simulink model "simulateController"  (R2022a)
settings: Solver=ode5  StartTime=0.0  StopTime=480  RelTol=1e-3
values from neighbouring files (symbols this model uses):
  ss_d = c2d(bicycle, opts.Ts_mpc)    [readySimulation.m]
undefined symbols (not defined in the file or in its folder): A_full, B_full, C_full, lb_u_full, lb_x_full, opts, QstructInitial, R_full, R_full_zeros, ub_u_full, ub_x_full
settings Model: PacingRate=0.350000  Creator=simonas  LastModifiedBy=simonas
settings HardwareCC: ProdBitPerLong=64  ProdHWDeviceType=Intel->x86-64 (Linux 64)
settings RTWCC: Description=Simulink Desktop Real-Time  SystemTargetFile=sldrt.tlc  TemplateMakefile=sldrt.tmf  RTWCompilerOptimization=on
settings CodeAppCC: MaxIdLength=95
settings SimulinkDesktopRealTimeCC: TargetLibSuffix=_sldrt.a  TargetPreCompLibLocation=C:\Program Files\MATLAB\R2022a\toolbox\sldrt\lib\win64

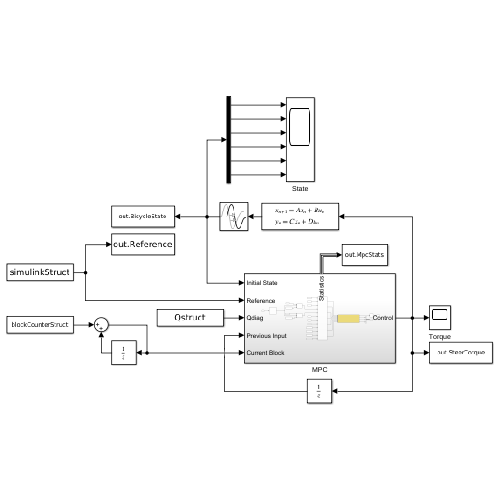
[thumbnail: Simulink's stored preview of the top-level diagram]
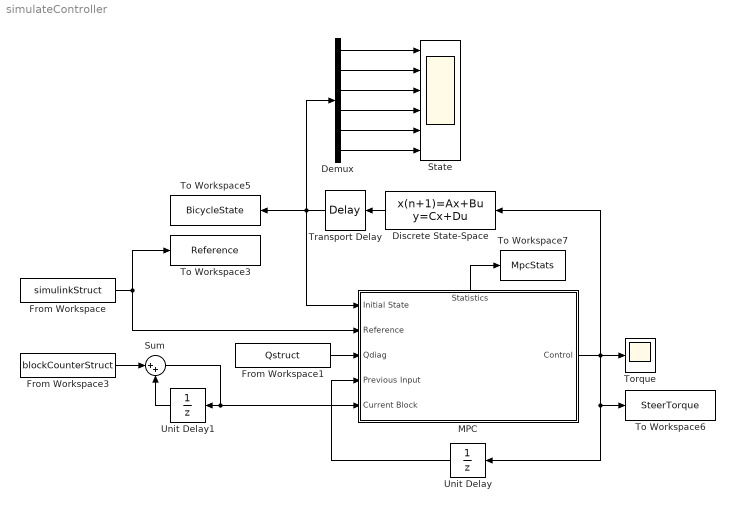
== system simulateController ==
  Demux : Demux  Outputs=6
  Discrete State-Space : DiscreteStateSpace  A=ss_d.A  B=ss_d.B  C=ss_d.C  D=ss_d.D  InitialCondition=[0; 0; 0; 0; 0; 0]  SampleTime=-1
  From Workspace : FromWorkspace  VariableName=simulinkStruct  SampleTime=opts.Ts_mpc  Interpolate=off  OutputAfterFinalValue=Cyclic repetition
  From Workspace1 : FromWorkspace  VariableName=Qstruct  SampleTime=opts.Ts_mpc  Interpolate=off  OutputAfterFinalValue=Cyclic repetition
  From Workspace3 : FromWorkspace  VariableName=blockCounterStruct  SampleTime=opts.Ts_mpc  Interpolate=off  OutputAfterFinalValue=Cyclic repetition
  MPC : Subsystem
      settings: PortSchema="{\"entries\":[{\"content\":{\"sides\":[{\"content\":{\"connectorIds\":[\"In1\",\"In2\",\"In3\",\"In4\",\"In5\"]},\"type\":\"ConnectorPlacement.EquallySpacedRectSide\",\"uuid\":\"837940b0-492f-49e7-ad78-2f53a96cfdb0\"},{\"content\":{\"connectorIds\":[\"Out1\"],\"side\":\"RIGHT\"},\"type\":\"ConnectorPlacement.EquallySpacedRectSide\",\"uuid\":\"0b454771-57c7-4798-97e4-6e41a25b36dc\"},{\"content\":{\"connectorIds\":[\"Out2\"],\"side\":\"TOP\"},\"type\":\"ConnectorPlacement.EquallySpacedRectSide\",\"uuid\":\"d0d77e63-f0c6-441e-9a4a-b6dfb0057ad2\"},{\"content\":{\"connectorIds\":[],\"side\":\"BOTTOM\"},\"type\":\"ConnectorPlacement.EquallySpacedRectSide\",\"uuid\":\"b6921f02-8dc3-4ff1-8cb0-61ac83bc5ab1\"}]},\"type\":\"ConnectorPlacement.EquallySpacedConnector\",\"uuid\":\"6905a0a5-9fd3-4ab9-9143-61679843e617\"}],\"packageUris\":[\"http://schema.mathworks.com/mf0/Connector/R2020b\"],\"version\":\"1.0\"}"
  State : Scope  NumInputPorts=6
  Sum : Sum  Inputs=|++
  To Workspace3 : ToWorkspace  VariableName=Reference  SaveFormat=Timeseries  SampleTime=-1
  To Workspace5 : ToWorkspace  VariableName=BicycleState  SaveFormat=Timeseries  SampleTime=-1
  To Workspace6 : ToWorkspace  VariableName=SteerTorque  SaveFormat=Timeseries  SampleTime=-1
  To Workspace7 : ToWorkspace  VariableName=MpcStats  SaveFormat=Timeseries  SampleTime=-1
  Torque : Scope
  Transport Delay : TransportDelay  DelayTime=0.1  InitialOutput=[0; 0; 0; 0; 0; 0]
  Unit Delay : UnitDelay  SampleTime=opts.Ts_mpc  HasFrameUpgradeWarning=on
  Unit Delay1 : UnitDelay  InitialCondition=1  SampleTime=opts.Ts_mpc  HasFrameUpgradeWarning=on
  wires:
  Discrete State-Space/1 -> Transport Delay/1
  MPC/1(Control) -> To Workspace6/1, Unit Delay/1, Torque/1, Discrete State-Space/1
  From Workspace/1 -> To Workspace3/1, MPC/2(Reference)
  From Workspace1/1 -> MPC/3(Qdiag)
  MPC/2(Statistics) -> To Workspace7/1
  Unit Delay/1 -> MPC/4(Previous Input)
  Demux/1 -> State/1
  Demux/3 -> State/3
  Demux/4 -> State/4
  Demux/2 -> State/2
  Demux/5 -> State/5
  Demux/6 -> State/6
  Sum/1 -> MPC/5(Current Block), Unit Delay1/1
  Transport Delay/1 -> Demux/1, To Workspace5/1, MPC/1(Initial State)
  From Workspace3/1 -> Sum/1
  Unit Delay1/1 -> Sum/2

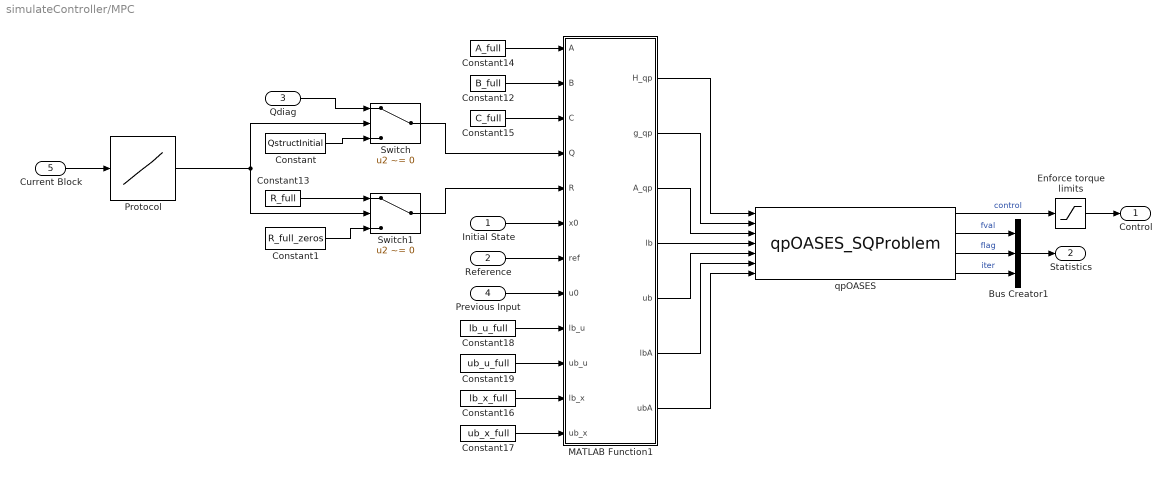
== system simulateController/MPC ==
  Initial State : Inport
  Reference : Inport  Port=2
  Qdiag : Inport  Port=3
  Previous Input : Inport  Port=4
  Current Block : Inport  Port=5
  Bus Creator1 : BusCreator  Inputs=3
  Constant : Constant  Value=QstructInitial
  Constant1 : Constant  Value=R_full_zeros  SampleTime=opts.Ts_mpc
  Constant12 : Constant  Value=B_full  SampleTime=opts.Ts_mpc
  Constant13 : Constant  Value=R_full  SampleTime=opts.Ts_mpc
  Constant14 : Constant  Value=A_full  SampleTime=opts.Ts_mpc
  Constant15 : Constant  Value=C_full  SampleTime=opts.Ts_mpc
  Constant16 : Constant  Value=lb_x_full  SampleTime=opts.Ts_mpc
  Constant17 : Constant  Value=ub_x_full  SampleTime=opts.Ts_mpc
  Constant18 : Constant  Value=lb_u_full  SampleTime=opts.Ts_mpc
  Constant19 : Constant  Value=ub_u_full  SampleTime=opts.Ts_mpc
  Enforce torque limits : Saturate  UpperLimit=opts.steerTorqueLim  LowerLimit=-opts.steerTorqueLim
  MATLAB Function1 : MATLAB Function  TreatAsAtomicUnit=on  SystemSampleTime=opts.Ts_mpc  VariantControl=Choice
  Protocol : Lookup_n-D  NumberOfTableDimensions=1  BreakpointsForDimension1=opts.lookupBreakpoints  Table=opts.lookupValues  InternalRulePriority=Speed  RndMeth=Simplest
  Switch : Switch  Criteria=u2 ~= 0  SaturateOnIntegerOverflow=off  InputSameDT=off
  Switch1 : Switch  Criteria=u2 ~= 0  SaturateOnIntegerOverflow=off  InputSameDT=off
  qpOASES : S-Function  FunctionName=qpOASES_SQProblem  SFunctionDeploymentMode=off  EnableBusSupport=off
  Control : Outport
  Statistics : Outport  Port=2
  wires:
  Enforce torque limits/1 -> Control/1
  Constant12/1 -> MATLAB Function1/2(B)
  Constant18/1 -> MATLAB Function1/9(lb_u)
  MATLAB Function1/1(H_qp) -> qpOASES/1
  Constant16/1 -> MATLAB Function1/11(lb_x)
  Constant19/1 -> MATLAB Function1/10(ub_u)
  Constant17/1 -> MATLAB Function1/12(ub_x)
  Bus Creator1/1 -> Statistics/1
  qpOASES/4 -> Bus Creator1/3  "iter"
  qpOASES/2 -> Bus Creator1/1  "fval"
  MATLAB Function1/3(A_qp) -> qpOASES/3
  Reference/1 -> MATLAB Function1/7(ref)
  qpOASES/3 -> Bus Creator1/2  "flag"
  MATLAB Function1/4(lb) -> qpOASES/4
  MATLAB Function1/2(g_qp) -> qpOASES/2
  Constant14/1 -> MATLAB Function1/1(A)
  MATLAB Function1/5(ub) -> qpOASES/5
  MATLAB Function1/7(ubA) -> qpOASES/7
  Constant15/1 -> MATLAB Function1/3(C)
  MATLAB Function1/6(lbA) -> qpOASES/6
  Previous Input/1 -> MATLAB Function1/8(u0)
  Initial State/1 -> MATLAB Function1/6(x0)
  qpOASES/1 -> Enforce torque limits/1  "control"
  Current Block/1 -> Protocol/1
  Switch/1 -> MATLAB Function1/4(Q)
  Qdiag/1 -> Switch/1
  Switch1/1 -> MATLAB Function1/5(R)
  Constant13/1 -> Switch1/1
  Protocol/1 -> Switch1/2, Switch/2
  Constant/1 -> Switch/3
  Constant1/1 -> Switch1/3

== matlab function simulateController/MPC/MATLAB Function1 ==
  data: H_qp output; g_qp output; A input; A_qp output; B input; C input; Q input; R input; x0 input; ref input; u0 input; lb_u input; ub_u input; lb_x input; ub_x input; lb output; ub output; lbA output; ubA output
function [H_qp, g_qp, A_qp, lb, ub, lbA, ubA] = fcn(A, B, C, Q, R, x0, ref, u0, lb_u, ub_u, lb_x, ub_x) %#codegen

temp = B' .* Q';
H = temp * B + R;

A_qp = B(:);
H_qp = H(:);
g_qp = [temp * A, ...
        -temp, ...
        temp * C] * [x0; ref; u0];

temp = - A * x0 - C * u0;

lb = lb_u;
ub = ub_u;
lbA = lb_x + temp;
ubA = ub_x + temp;
